simulink library "cmg_model_lib"  (R2018b)
settings: Solver=VariableStepAuto  StartTime=0.0  StopTime=10.0  RelTol=1e-3
undefined symbols (not defined in the file or in its folder): Km, simParams
settings Model: Creator=colem  LastModifiedBy=colem
settings SFSimCC: SimUseLocalCustomCode=off
settings RTWCC: RTWUseLocalCustomCode=off

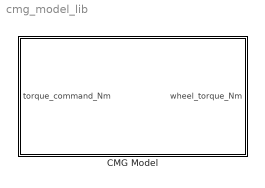
== system cmg_model_lib ==
  "CMG Model " : Subsystem

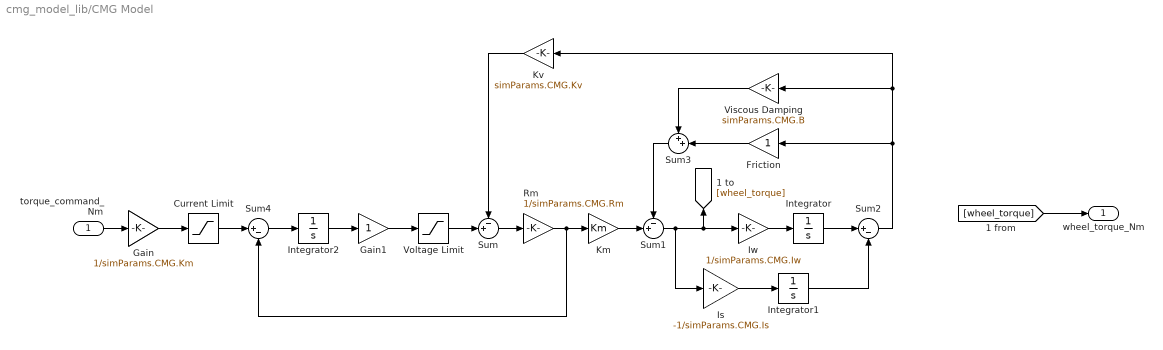
== system cmg_model_lib/CMG Model  ==
  torque_command_Nm : Inport
  Current Limit : Saturate  UpperLimit=simParams.CMG.current_limit  LowerLimit=-simParams.CMG.current_limit
  Friction : Gain
  Gain : Gain  Gain=1/simParams.CMG.Km
  Gain1 : Gain
  Integrator : Integrator
  Integrator1 : Integrator
  Integrator2 : Integrator
  Is : Gain  Gain=-1/simParams.CMG.Is
  Iw : Gain  Gain=1/simParams.CMG.Iw
  Km : Gain  Gain=Km
  Kv : Gain  Gain=simParams.CMG.Kv
  Rm : Gain  Gain=1/simParams.CMG.Rm
  Sum : Sum  Inputs=-+|
  Sum1 : Sum  Inputs=-+|
  Sum2 : Sum  Inputs=|+-
  Sum3 : Sum  Inputs=++|
  Sum4 : Sum  Inputs=|+-
  Viscous Damping : Gain  Gain=simParams.CMG.B
  Voltage Limit : Saturate  UpperLimit=simParams.CMG.voltage_limit  LowerLimit=-simParams.CMG.voltage_limit
  wheel_torque_Nm : Outport
  wires:
  Voltage Limit/1 -> Sum/2
  Is/1 -> Integrator1/1
  Integrator1/1 -> Sum2/2
  Sum3/1 -> Sum1/1
  Friction/1 -> Sum3/2
  Sum1/1 -> Is/1, Iw/1, [wheel_torque]
  Integrator/1 -> Sum2/1
  Sum2/1 -> Viscous Damping/1, Kv/1, Friction/1
  Kv/1 -> Sum/1
  Viscous Damping/1 -> Sum3/1
  Sum/1 -> Rm/1
  Km/1 -> Sum1/2
  Iw/1 -> Integrator/1
  Rm/1 -> Sum4/2, Km/1
  Current Limit/1 -> Sum4/1
  Gain/1 -> Current Limit/1
  torque_command_Nm/1 -> Gain/1
  Sum4/1 -> Integrator2/1
  Integrator2/1 -> Gain1/1
  Gain1/1 -> Voltage Limit/1
  [wheel_torque] -> wheel_torque_Nm/1
